simulink model "Prac_6"  (R2022b)
settings: Solver=VariableStepAuto  StartTime=0.0  StopTime=10.0  RelTol=1e-3
model workspace (MAT data in the model file):
  A = 10
  C = 10
  GCelcius = Simulink.Parameter
  GCelcius.Value = 30
  GCelcius.DataType = 'auto'
  GCelcius.Complexity = 'real'
  GCelcius.Dimensions = [1 1]
  GradoCelc = 27
  GradosCelcius = 1
  K = 20
  m = 5
  sig = -1
  x = 5
  y = 2
settings Model: Creator=cesar  LastModifiedBy=cesar

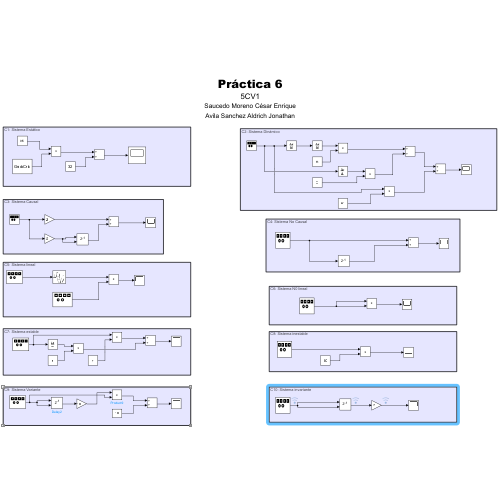
[thumbnail: Simulink's stored preview of the top-level diagram]
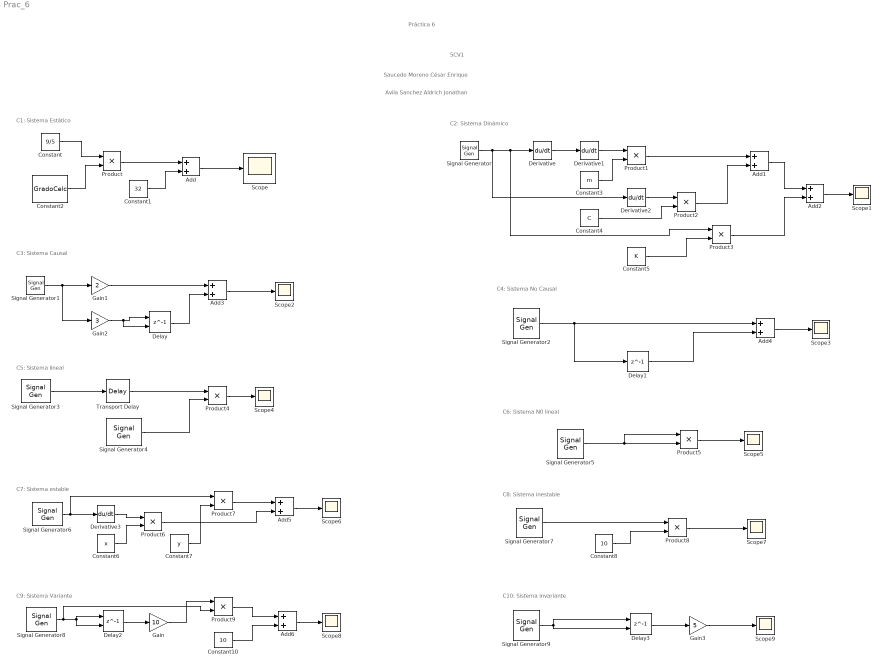
== system Prac_6 ==
  note: C9: Sistema Variante
  note: C8: Sistema inestable
  note: C7: Sistema estable
  note: C5: Sistema lineal
  note: C4: Sistema No Causal
  note: C3: Sistema Causal
  note: C2: Sistema Dinámico
  note: C1: Sistema Estático
  note: 5CV1
  note: Avila Sanchez Aldrich Jonathan
  note: Saucedo Moreno César Enrique
  note: Práctica 6
  note: C6: Sistema N0 lineal
  note: C10: Sistema invariante
  Add{,1..6} (7 alike) : Sum
  Constant : Constant  Value=9/5
  Constant1 : Constant  Value=32
  Constant10 : Constant  Value=10
  Constant2 : Constant  Value=GradoCelc
  Constant3 : Constant  Value=m
  Constant4 : Constant  Value=C
  Constant5 : Constant  Value=K
  Constant6 : Constant  Value=x
  Constant7 : Constant  Value=y
  Constant8 : Constant  Value=10
  Delay : Delay  DelayLength=1  InitialConditionSource=Input port  InitialCondition=0  InputProcessing=Columns as channels (frame based)
      settings: InputPortMap=u0,p4
  Delay1 : Delay  DelayLength=1  DelayLengthUpperLimit=-2  InitialCondition=0  InputProcessing=Columns as channels (frame based)  UseCircularBuffer=on  SampleTime=1
  Delay2 : Delay  DelayLength=1  InitialConditionSource=Input port  InitialCondition=0  InputProcessing=Columns as channels (frame based)
      settings: InputPortMap=u0,p4
  Delay3 : Delay  DelayLength=1  InitialConditionSource=Input port  InitialCondition=0  InputProcessing=Columns as channels (frame based)
      settings: InputPortMap=u0,p4
  Derivative{,1..3} (4 alike) : Derivative
  Gain : Gain  Gain=10
  Gain1 : Gain  Gain=2
  Gain2 : Gain  Gain=3
  Gain3 : Gain  Gain=5
  Product{,1..9} (10 alike) : Product
  Scope{,1..9} (10 alike) : Scope
  Signal Generator : SignalGenerator  Units=rad/sec
  Signal Generator1 : SignalGenerator  WaveForm=square  Units=rad/sec
  Signal Generator2 : SignalGenerator  WaveForm=sawtooth  Units=rad/sec
  Signal Generator3 : SignalGenerator  WaveForm=square  Units=rad/sec
  Signal Generator4 : SignalGenerator  Amplitude=10  Units=rad/sec
  Signal Generator5 : SignalGenerator  WaveForm=square  Units=rad/sec
  Signal Generator6 : SignalGenerator  Units=rad/sec
  Signal Generator7 : SignalGenerator  WaveForm=square  Amplitude=2  Units=rad/sec
  Signal Generator8 : SignalGenerator  Units=rad/sec
  Signal Generator9 : SignalGenerator  Amplitude=2  Units=rad/sec
  Transport Delay : TransportDelay  DelayTime=2  InitialOutput=sig
  wires:
  Constant/1 -> Product/1
  Product/1 -> Add/1
  Constant1/1 -> Add/2
  Add/1 -> Scope/1
  Constant2/1 -> Product/2
  Signal Generator/1 -> Derivative2/1, Product3/1, Derivative/1
  Derivative/1 -> Derivative1/1
  Derivative1/1 -> Product1/1
  Constant3/1 -> Product1/2
  Derivative2/1 -> Product2/1
  Constant4/1 -> Product2/2
  Constant5/1 -> Product3/2
  Product1/1 -> Add1/1
  Product2/1 -> Add1/2
  Product3/1 -> Add2/2
  Add1/1 -> Add2/1
  Add2/1 -> Scope1/1
  Signal Generator1/1 -> Gain2/1, Gain1/1
  Gain2/1 -> Delay/2, Delay/1
  Gain1/1 -> Add3/1
  Delay/1 -> Add3/2
  Add3/1 -> Scope2/1
  Delay1/1 -> Add4/2
  Signal Generator2/1 -> Add4/1, Delay1/1
  Add4/1 -> Scope3/1
  Product4/1 -> Scope4/1
  Signal Generator4/1 -> Product4/2
  Signal Generator3/1 -> Transport Delay/1
  Transport Delay/1 -> Product4/1
  Signal Generator5/1 -> Product5/2, Product5/1
  Product5/1 -> Scope5/1
  Signal Generator6/1 -> Product7/1, Derivative3/1
  Constant6/1 -> Product6/2
  Derivative3/1 -> Product6/1
  Constant7/1 -> Product7/2
  Product7/1 -> Add5/1
  Product6/1 -> Add5/2
  Add5/1 -> Scope6/1
  Signal Generator7/1 -> Product8/1
  Constant8/1 -> Product8/2
  Product8/1 -> Scope7/1
  Signal Generator8/1 -> Product9/2, Delay2/2, Delay2/1
  Delay2/1 -> Gain/1
  Gain/1 -> Product9/1
  Product9/1 -> Add6/1
  Constant10/1 -> Add6/2
  Add6/1 -> Scope8/1
  Signal Generator9/1 -> Delay3/1, Delay3/2
  Delay3/1 -> Gain3/1
  Gain3/1 -> Scope9/1
